simulink model "PassengerCar"  (R2019b)
settings: Solver=ode1  StartTime=0  StopTime=25  FixedStep=1.0000000000000000e-003  RelTol=1e-3
InitFcn:
  | sampleTime = str2double(get_param(bdroot, 'FixedStep'));
undefined symbols (not defined in the file or in its folder): AccPedalPos, BrakePedalPos, BrakeSwitch, DiscIntNeverNeededParam, DYNA4, EngSpd, IgnitionSwitch, InitialGear, InitialSpeed, IntendedEngTrq, LeftIndicator, MainBrakePress, MaxGear, MDL, MinGear, RefAcc, RefLane, RefLatPos, RefPath, RefPathCurv, RefSpd, RefSpdPreview, RefSpdRetrospect, RightIndicator, SteeringWheelAng, SteeringWheelTrq, UserDefinedRefValue, vm_const
libraries: UtilitiesLibrary x31, simulink x18, WheelSystemModules x13, LongitudinalControllerModules x13, LateralControllerModules x7, AnimationBusselectorModules x5, EnvironmentModules x5, BasicEngineControlModules x5, MiscellaneousControlModules x5, Animation3Modules x4, AuxiliariesModules x4, TireModules x4
(part 5 of 39)

== system PassengerCar/Traffic/TrafficOutputs ==
  Distance : Constant  Value=1000
  Distance1 : Constant  Value=0
  DistanceToVehicleOutput : Subsystem  Tag=TESIS DYNAware Interface Block  mask{NeedsUpdate=off, SignalInfo=|}
      mask SignalInfo=|
      | {
      |   "Version": "4.6",
      |   "MuxedOutputBusName": "Traffic",
      |   "MuxedInputBusName": "input",
      |   "MuxedInputSelected": false,
      |   "MuxedOutputSelected": true,
      |   "SignalData": [
      |     {
      |       "initialValue": "0.0",
      |       "name": "LeftAdjacentLaneFrontalDist[m]",
      |       "comment": "Distance of VuT to next frontal traffic object on left adjacent lane",
      |       "minString": "",
      |       "maxString": "",
      |       "width": 1,
      |       "dataType": 0,
      |       "signalType": 0,
      |       "createSignal": false,
      |       "outputName": "DistancesToVehicle.LeftAdjacentLaneFrontalDist[m]",
      |       "generateSignalAccessBlock": false,
      |       "accessId": "$(parentId).$(blockName).$(outputName)"
      |     },
      |     {
      |       "initialValue": "0.0",
      |       "name": "LeftAdjacentLaneRearDist[m]",
      |       "comment": "Distance of VuT to next rear traffic object on left adjacent lane",
      |       "minString": "",
      |       "maxString": "",
      |       "width": 1,
      |       "dataType": 0,
      |       "signalType": 0,
      |       "createSignal": false,
      |       "outputName": "DistancesToVehicle.LeftAdjacentLaneRearDist[m]",
      |       "generateSignalAccessBlock": false,
      |       "accessId": "$(parentId).$(blockName).$(outputName)"
      |     },
      |     {
      |       "initialValue": "0.0",
      |       "name": "MyLaneFrontalDist[m]",
      |       "comment": "Distance of VuT to next frontal traffic object on the same lane",
      |       "minString": "",
      |       "maxString": "",
      |       "width": 1,
      |       "dataType": 0,
      |       "signalType": 0,
      |       "createSignal": false,
      |       "outputName": "DistancesToVehicle.MyLaneFrontalDist[m]",
      |       "generateSignalAccessBlock": false,
      |       "accessId": "$(parentId).$(blockName).$(outputName)"
      |     },
      |     {
      |       "initialValue": "0.0",
      |       "name": "MyLaneRearDist[m]",
      |       "comment": "Distance of VuT to next rear traffic object on the same lane",
      |       "minString": "",
      |       "maxString": "",
      |       "width": 1,
      |       "dataType": 0,
      |       "signalType": 0,
      |       "createSignal": false,
      |       "outputName": "DistancesToVehicle.MyLaneRearDist[m]",
      |       "generateSignalAccessBlock": false,
      |       "accessId": "$(parentId).$(blockName).$(outputName)"
      |     },
      |     {
      |       "initialValue": "0.0",
      |       "name": "RightAdjacentLaneFrontalDist[m]",
      |       "comment": "Distance of VuT to next frontal traffic object on right adjacent lane",
      |       "minString": "",
      |       "maxString": "",
      |       "width": 1,
      |       "dataType": 0,
      |       "signalType": 0,
      |       "createSignal": false,
      |       "outputName": "DistancesToVehicle.RightAdjacentLaneFrontalDist[m]",
      |       "generateSignalAccessBlock": false,
      |       "accessId": "$(parentId).$(blockName).$(outputName)"
      |     },
      |     {
      |       "initialValue": "0.0",
      |       "name": "RightAdjacentLaneRearDist[m]",
      |       "comment": "Distance of VuT to next rear traffic object on right adjacent lane",
      |       "minString": "",
      |       "maxString": "",
      |       "width": 1,
      |       "dataType": 0,
      |       "signalType": 0,
      |       "createSignal": false,
      |       "outputName": "DistancesToVehicle.RightAdjacentLaneRearDist[m]",
      |       "generateSignalAccessBlock": false,
      |       "accessId": "$(parentId).$(blockName).$(outputName)"
      |     },
      |     {
      |       "initialValue": "0.0",
      |       "name": "LeftAdjacentLaneFrontalSpd[m/s]",
      |       "comment": "Longitudinal speed of next frontal traffic object on left adjacent lane",
      |       "minString": "",
      |       "maxString": "",
      |       "width": 1,
      |       "dataType": 0,
      |       "signalType": 0,
      |       "createSignal": false,
      |       "outputName": "AdjacentObjectsSpeeds.LeftAdjacentLaneFrontalSpd[m/s]",
      |       "generateSignalAccessBlock": false,
      |       "accessId": "$(parentId).$(blockName).$(outputName)"
      |     },
      |     {
      |       "initialValue": "0.0",
      |       "name": "LeftAdjacentLaneRearSpd[m/s]",
      |       "comment": "Longitudinal speed of next rear traffic object on left adjacent lane",
      |       "minString": "",
      |       "maxString": "",
      |       "width": 1,
      |       "dataType": 0,
      |       "signalType": 0,
      |       "createSignal": false,
      |       "outputName": "AdjacentObjectsSpeeds.LeftAdjacentLaneRearSpd[m/s]",
      |       "generateSignalAccessBlock": false,
      |       "accessId": "$(parentId).$(blockName).$(outputName)"
      |     },
      |     {
      |       "initialValue": "0.0",
      |       "name": "MyLaneFrontalSpd[m/s]",
      |       "comment": "Longitudinal speed of next frontal traffic object on the same lane",
      |       "minString": "",
      |       "maxString": "",
      |       "width": 1,
      |       "dataType": 0,
      |       "signalType": 0,
      |       "createSignal": false,
      |       "outputName": "AdjacentObjectsSpeeds.MyLaneFrontalSpd[m/s]",
      |       "generateSignalAccessBlock": false,
      |       "accessId": "$(parentId).$(blockName).$(outputName)"
      |     },
      |     {
      |       "initialValue": "0.0",
      |       "name": "MyLaneRearSpd[m/s]",
      |       "comment": "Longitudinal speed of next rear traffic object on the same lane",
      |       "minString": "",
      |       "maxString": "",
      |       "width": 1,
      |       "dataType": 0,
      |       "signalType": 0,
      |       "createSignal": false,
      |       "outputName": "AdjacentObjectsSpeeds.MyLaneRearSpd[m/s]",
      |       "generateSignalAccessBlock": false,
      |       "accessId": "$(parentId).$(blockName).$(outputName)"
      |     },
      |     {
      |       "initialValue": "0.0",
      |       "name": "RightAdjacentLaneFrontalSpd[m/s]",
      |       "comment": "Longitudinal speed of next frontal traffic object on right adjacent lane",
      |       "minString": "",
      |       "maxString": "",
      |       "width": 1,
      |       "dataType": 0,
      |       "signalType": 0,
      |       "createSignal": false,
      |       "outputName": "AdjacentObjectsSpeeds.RightAdjacentLaneFrontalSpd[m/s]",
      |       "generateSignalAccessBlock": false,
      |       "accessId": "$(parentId).$(blockName).$(outputName)"
      |     },
      |     {
      |       "initialValue": "0.0",
      |       "name": "RightAdjacentLaneRearSpd[m/s]",
      |       "comment": "Longitudinal speed of next rear traffic object on right adjacent lane",
      |       "minString": "",
      |       "maxString": "",
      |       "width": 1,
      |       "dataType": 0,
      |       "signalType": 0,
      |       "createSignal": false,
      |       "outputName": "AdjacentObjectsSpeeds.RightAdjacentLaneRearSpd[m/s]",
      |       "generateSignalAccessBlock": false,
      |       "accessId": "$(parentId).$(blockName).$(outputName)"
      |     }
      |   ]
      | }
      mask prompts: NeedsUpdate "Specify, if subsystem content needs to be updated"; SignalInfo "Signal Info (json)"
      mask help: DYNA4 Interface Block Version 4.6
      mask init:
      | blockName = get_param(gcbh, 'Name');
      | parentId = DYNA4.ModelHandling.AccessID.getFromHierarchy(gcbh);
      | TD.InterfaceBlock.ModelCallbacks.GenerateContent(gcb);
      settings: DeleteFcn=TD.InterfaceBlock.ModelCallbacks.CloseGUI( gcbh );  NameChangeFcn=TD.InterfaceBlock.ModelCallbacks.BlockRenamedHandler(gcbh);  OpenFcn=TD.InterfaceBlock.ModelCallbacks.OpenGUI( gcbh );  CloseFcn=TD.InterfaceBlock.ModelCallbacks.CloseGUI( gcbh );
      mask Display:
      | image('InterfaceBlock.png','center');
      | port_label('input',1, 'LeftAdjacentLaneFrontalDist[m]');
      | port_label('input',2, 'LeftAdjacentLaneRearDist[m]');
      | port_label('input',3, 'MyLaneFrontalDist[m]');
      | port_label('input',4, 'MyLaneRearDist[m]');
      | port_label('input',5, 'RightAdjacentLaneFrontalDist[m]');
      | port_label('input',6, 'RightAdjacentLaneRearDist[m]');
      | port_label('input',7, 'LeftAdjacentLaneFrontalSpd[m/s]');
      | port_label('input',8, 'LeftAdjacentLaneRearSpd[m/s]');
      | port_label('input',9, 'MyLaneFrontalSpd[m/s]');
      | port_label('input',10, 'MyLaneRearSpd[m/s]');
      | port_label('input',11, 'RightAdjacentLaneFrontalSpd[m/s]');
      | port_label('input',12, 'RightAdjacentLaneRearSpd[m/s]');
      | port_label('output',1, 'Traffic');
  Traffic : Outport  VectorParamsAs1DForOutWhenUnconnected=off
  wires:
  Distance1/1 -> DistanceToVehicleOutput/12(RightAdjacentLaneRearSpd[m/s]___UNIQUE_1), DistanceToVehicleOutput/11(RightAdjacentLaneFrontalSpd[m/s]___UNIQUE_1), DistanceToVehicleOutput/10(MyLaneRearSpd[m/s]___UNIQUE_1), DistanceToVehicleOutput/7(LeftAdjacentLaneFrontalSpd[m/s]___UNIQUE_1), DistanceToVehicleOutput/8(LeftAdjacentLaneRearSpd[m/s]___UNIQUE_1), DistanceToVehicleOutput/9(MyLaneFrontalSpd[m/s]___UNIQUE_1)
  Distance/1 -> DistanceToVehicleOutput/5(RightAdjacentLaneFrontalDist[m]___UNIQUE_1), DistanceToVehicleOutput/6(RightAdjacentLaneRearDist[m]___UNIQUE_1), DistanceToVehicleOutput/4(MyLaneRearDist[m]___UNIQUE_1), DistanceToVehicleOutput/3(MyLaneFrontalDist[m]___UNIQUE_1), DistanceToVehicleOutput/2(LeftAdjacentLaneRearDist[m]___UNIQUE_1), DistanceToVehicleOutput/1(LeftAdjacentLaneFrontalDist[m]___UNIQUE_1)
  DistanceToVehicleOutput/1(Traffic___UNIQUE_1) -> Traffic/1

== system PassengerCar/Trailer/DynaComponentInfo ==

== system PassengerCar/Vehicle/Auxiliaries ==
  fromCTRL : Inport
  fromDrivetrain : Inport  Port=2
  fromElectricalSystem : Inport  Port=3
  fromEngine : Inport  Port=4
  AuxiliariesOutput : Subsystem  Tag=TESIS DYNAware Interface Block  mask{NeedsUpdate=off, SignalInfo=|}
      mask SignalInfo=|
      | {
      |   "Version": "4.6",
      |   "MuxedOutputBusName": "Auxiliaries",
      |   "MuxedInputBusName": "input",
      |   "MuxedInputSelected": false,
      |   "MuxedOutputSelected": true,
      |   "SignalData": [
      |     {
      |       "initialValue": "0.0",
      |       "name": "GeneratorCurr[A]",
      |       "comment": "",
      |       "minString": "",
      |       "maxString": "",
      |       "width": 1,
      |       "dataType": 0,
      |       "signalType": 0,
      |       "createSignal": false,
      |       "outputName": "GeneratorCurr[A]",
      |       "generateSignalAccessBlock": false,
      |       "accessId": "$(parentId).$(blockName).$(outputName)"
      |     },
      |     {
      |       "initialValue": "0.0",
      |       "name": "GeneratorTrq[Nm]",
      |       "comment": "",
      |       "minString": "",
      |       "maxString": "",
      |       "width": 1,
      |       "dataType": 0,
      |       "signalType": 0,
      |       "createSignal": false,
      |       "outputName": "GeneratorTrq[Nm]",
      |       "generateSignalAccessBlock": false,
      |       "accessId": "$(parentId).$(blockName).$(outputName)"
      |     },
      |     {
      |       "initialValue": "0.0",
      |       "name": "GeneratorInrt[kgm^2]",
      |       "comment": "",
      |       "minString": "",
      |       "maxString": "",
      |       "width": 1,
      |       "dataType": 0,
      |       "signalType": 0,
      |       "createSignal": false,
      |       "outputName": "GeneratorInrt[kgm^2]",
      |       "generateSignalAccessBlock": false,
      |       "accessId": "$(parentId).$(blockName).$(outputName)"
      |     },
      |     {
      |       "initialValue": "0.0",
      |       "name": "StarterCurr[A]",
      |       "comment": "",
      |       "minString": "",
      |       "maxString": "",
      |       "width": 1,
      |       "dataType": 0,
      |       "signalType": 0,
      |       "createSignal": false,
      |       "outputName": "StarterCurr[A]",
      |       "generateSignalAccessBlock": false,
      |       "accessId": "$(parentId).$(blockName).$(outputName)"
      |     },
      |     {
      |       "initialValue": "0.0",
      |       "name": "StarterTrq[Nm]",
      |       "comment": "",
      |       "minString": "",
      |       "maxString": "",
      |       "width": 1,
      |       "dataType": 0,
      |       "signalType": 0,
      |       "createSignal": false,
      |       "outputName": "StarterTrq[Nm]",
      |       "generateSignalAccessBlock": false,
      |       "accessId": "$(parentId).$(blockName).$(outputName)"
      |     },
      |     {
      |       "initialValue": "0.0",
      |       "name": "StarterInrt[kgm**2]",
      |       "comment": "",
      |       "minString": "",
      |       "maxString": "",
      |       "width": 1,
      |       "dataType": 0,
      |       "signalType": 0,
      |       "createSignal": false,
      |       "outputName": "StarterInrt[kgm**2]",
      |       "generateSignalAccessBlock": false,
      |       "accessId": "$(parentId).$(blockName).$(outputName)"
      |     }
      |   ]
      | }
      mask prompts: NeedsUpdate "Specify, if subsystem content needs to be updated"; SignalInfo "Signal Info (json)"
      mask help: DYNA4 Interface Block Version 4.6
      mask init:
      | blockName = get_param(gcbh, 'Name');
      | parentId = DYNA4.ModelHandling.AccessID.getFromHierarchy(gcbh);
      | TD.InterfaceBlock.ModelCallbacks.GenerateContent(gcb);
      settings: DeleteFcn=TD.InterfaceBlock.ModelCallbacks.CloseGUI( gcbh );  NameChangeFcn=TD.InterfaceBlock.ModelCallbacks.BlockRenamedHandler(gcbh);  OpenFcn=TD.InterfaceBlock.ModelCallbacks.OpenGUI( gcbh );  CloseFcn=TD.InterfaceBlock.ModelCallbacks.CloseGUI( gcbh );
      mask Display:
      | image('InterfaceBlock.png','center');
      | port_label('input',1, 'GeneratorCurr[A]');
      | port_label('input',2, 'GeneratorTrq[Nm]');
      | port_label('input',3, 'GeneratorInrt[kgm^2]');
      | port_label('input',4, 'StarterCurr[A]');
      | port_label('input',5, 'StarterTrq[Nm]');
      | port_label('input',6, 'StarterInrt[kgm**2]');
      | port_label('output',1, 'Auxiliaries');
  DynaComponentInfo : Subsystem  Tag=DynaComponentInfo
      mask init:
      | data= get_param(gcb, 'UserData');
      settings: OpenFcn=DYNA4.ModelHandling.Component.ShowEditComponentInformationDialog(gcb);
      mask Display: disp(['Type = ', data.type, '\nGroup = ', data.group, '\nName = ', data.name ])
  Generator : Subsystem
  GeneratorTemp [K] : Constant  Value=273+80
  InputFromCTRL : Subsystem  Tag=TESIS DYNAware Interface Block  mask{NeedsUpdate=off, SignalInfo=|}
      mask SignalInfo=|
      | {
      |   "Version": "4.6",
      |   "MuxedOutputBusName": "Ctrl",
      |   "MuxedInputBusName": "fromCTRL",
      |   "MuxedInputSelected": true,
      |   "MuxedOutputSelected": false,
      |   "SignalData": [
      |     {
      |       "initialValue": "0.0",
      |       "name": "CTRL.LongitudinalControl.StarterSwitch[0;1]",
      |       "comment": "Engine starter switch",
      |       "minString": "",
      |       "maxString": "",
      |       "width": 1,
      |       "dataType": 0,
      |       "signalType": 0,
      |       "createSignal": false,
      |       "outputName": "StarterSwitch[0;1]",
      |       "generateSignalAccessBlock": false,
      |       "accessId": "$(parentId).$(blockName).$(outputName)"
      |     },
      |     {
      |       "initialValue": "0.0",
      |       "name": "CTRL.EnvironmentalConditions.AmbTemp[K]",
      |       "comment": "",
      |       "minString": "",
      |       "maxString": "",
      |       "width": 1,
      |       "dataType": 0,
      |       "signalType": 0,
      |       "createSignal": false,
      |       "outputName": "AmbTemp[K]",
      |       "generateSignalAccessBlock": false,
      |       "accessId": "$(parentId).$(blockName).$(outputName)"
      |     }
      |   ]
      | }
      mask prompts: NeedsUpdate "Specify, if subsystem content needs to be updated"; SignalInfo "Signal Info (json)"
      mask help: DYNA4 Interface Block Version 4.6
      mask init:
      | blockName = get_param(gcbh, 'Name');
      | parentId = DYNA4.ModelHandling.AccessID.getFromHierarchy(gcbh);
      | TD.InterfaceBlock.ModelCallbacks.GenerateContent(gcb);
      settings: DeleteFcn=TD.InterfaceBlock.ModelCallbacks.CloseGUI( gcbh );  NameChangeFcn=TD.InterfaceBlock.ModelCallbacks.BlockRenamedHandler(gcbh);  OpenFcn=TD.InterfaceBlock.ModelCallbacks.OpenGUI( gcbh );  CloseFcn=TD.InterfaceBlock.ModelCallbacks.CloseGUI( gcbh );
      mask Display:
      | image('InterfaceBlock.png','center');
      | port_label('input',1, 'fromCTRL');
      | port_label('output',1, 'StarterSwitch[0;1]');
      | port_label('output',2, 'AmbTemp[K]');
  InputFromDrivetrain : Subsystem  Tag=TESIS DYNAware Interface Block  mask{NeedsUpdate=off, SignalInfo=|}
      mask SignalInfo=|
      | {
      |   "Version": "4.6",
      |   "MuxedOutputBusName": "output",
      |   "MuxedInputBusName": "fromDrivetrain",
      |   "MuxedInputSelected": true,
      |   "MuxedOutputSelected": false,
      |   "SignalData": {
      |     "initialValue": "0.0",
      |     "name": "DrivetrainPhysics.EngSpd[rad/s]",
      |     "comment": "",
      |     "minString": "",
      |     "maxString": "",
      |     "width": -1,
      |     "dataType": 0,
      |     "signalType": 0,
      |     "createSignal": false,
      |     "outputName": "EngSpd[rad/s]",
      |     "generateSignalAccessBlock": false,
      |     "accessId": "$(parentId).$(blockName).$(outputName)"
      |   }
      | }
      mask prompts: NeedsUpdate "Specify, if subsystem content needs to be updated"; SignalInfo "Signal Info (json)"
      mask help: DYNA4 Interface Block Version 4.6
      mask init:
      | blockName = get_param(gcbh, 'Name');
      | parentId = DYNA4.ModelHandling.AccessID.getFromHierarchy(gcbh);
      | TD.InterfaceBlock.ModelCallbacks.GenerateContent(gcb);
      settings: DeleteFcn=TD.InterfaceBlock.ModelCallbacks.CloseGUI( gcbh );  NameChangeFcn=TD.InterfaceBlock.ModelCallbacks.BlockRenamedHandler(gcbh);  OpenFcn=TD.InterfaceBlock.ModelCallbacks.OpenGUI( gcbh );  CloseFcn=TD.InterfaceBlock.ModelCallbacks.CloseGUI( gcbh );
      mask Display:
      | image('InterfaceBlock.png','center');
      | port_label('input',1, 'fromDrivetrain');
      | port_label('output',1, 'EngSpd[rad/s]');
  InputFromElectricalSystem : Subsystem  Tag=TESIS DYNAware Interface Block  mask{NeedsUpdate=off, SignalInfo=|}
      mask SignalInfo=|
      | {
      |   "Version": "4.6",
      |   "MuxedOutputBusName": "Powernet",
      |   "MuxedInputBusName": "fromPowernet",
      |   "MuxedInputSelected": true,
      |   "MuxedOutputSelected": false,
      |   "SignalData": [
      |     {
      |       "initialValue": "0.0",
      |       "name": "GeneratorVoltage[V]",
      |       "comment": "",
      |       "minString": "",
      |       "maxString": "",
      |       "width": 1,
      |       "dataType": 0,
      |       "signalType": 0,
      |       "createSignal": false,
      |       "outputName": "GeneratorVoltage[V]",
      |       "generateSignalAccessBlock": false,
      |       "accessId": "$(parentId).$(blockName).$(outputName)"
      |     },
      |     {
      |       "initialValue": "0.0",
      |       "name": "LowVoltageBattery.LowVoltageBatteryVoltage[V]",
      |       "comment": "",
      |       "minString": "",
      |       "maxString": "",
      |       "width": 1,
      |       "dataType": 0,
      |       "signalType": 0,
      |       "createSignal": false,
      |       "outputName": "LowVoltageBatteryVoltage[V]",
      |       "generateSignalAccessBlock": false,
      |       "accessId": "$(parentId).$(blockName).$(outputName)"
      |     },
      |     {
      |       "initialValue": "0.0",
      |       "name": "StarterVoltage[V]",
      |       "comment": "",
      |       "minString": "",
      |       "maxString": "",
      |       "width": 1,
      |       "dataType": 0,
      |       "signalType": 0,
      |       "createSignal": false,
      |       "outputName": "StarterVoltage[V]",
      |       "generateSignalAccessBlock": false,
      |       "accessId": "$(parentId).$(blockName).$(outputName)"
      |     }
      |   ]
      | }
      mask prompts: NeedsUpdate "Specify, if subsystem content needs to be updated"; SignalInfo "Signal Info (json)"
      mask help: DYNA4 Interface Block Version 4.6
      mask init:
      | blockName = get_param(gcbh, 'Name');
      | parentId = DYNA4.ModelHandling.AccessID.getFromHierarchy(gcbh);
      | TD.InterfaceBlock.ModelCallbacks.GenerateContent(gcb);
      settings: DeleteFcn=TD.InterfaceBlock.ModelCallbacks.CloseGUI( gcbh );  NameChangeFcn=TD.InterfaceBlock.ModelCallbacks.BlockRenamedHandler(gcbh);  OpenFcn=TD.InterfaceBlock.ModelCallbacks.OpenGUI( gcbh );  CloseFcn=TD.InterfaceBlock.ModelCallbacks.CloseGUI( gcbh );
      mask Display:
      | image('InterfaceBlock.png','center');
      | port_label('input',1, 'fromPowernet');
      | port_label('output',1, 'GeneratorVoltage[V]');
      | port_label('output',2, 'LowVoltageBatteryVoltage[V]');
      | port_label('output',3, 'StarterVoltage[V]');
  LoadResponse [s] : Constant  Value=3
  SimpleEnergyManagement : Subsystem
  Starter : Subsystem
  Terminator_6 : Terminator
  TraceMarker : UtilitiesLibrary/DYNA4 Trace Marker  Tag=DYNA4_TRACE_MARKER  SettingType=Standard  PrefixModelBlockID=on  PrefixRootSignalName=off  NamePattern='$(modelBlockID).$(rootSignalName)'
  Auxiliaries : Outport  VectorParamsAs1DForOutWhenUnconnected=off
  wires:
  InputFromElectricalSystem/3(StarterVoltage[V]___UNIQUE_1) -> Starter/1(StarterVoltage [V])
  Generator/1(Curr [A]) -> AuxiliariesOutput/1(GeneratorCurr[A]___UNIQUE_1)
  Generator/2(Trq [Nm]) -> AuxiliariesOutput/2(GeneratorTrq[Nm]___UNIQUE_1)
  Generator/3(Inrt [kgm**2]) -> AuxiliariesOutput/3(GeneratorInrt[kgm^2]___UNIQUE_1)
  InputFromCTRL/1(StarterSwitch[0;1]___UNIQUE_1) -> Starter/3(StarterSwitch [0;1]), SimpleEnergyManagement/1(StarterSwitch [0;1])
  Starter/1(StarterCurr [A]) -> AuxiliariesOutput/4(StarterCurr[A]___UNIQUE_1)
  InputFromCTRL/2(AmbTemp[K]___UNIQUE_1) -> Starter/4(Temp [K])
  LoadResponse [s]/1 -> Generator/4(LRTime [s])
  SimpleEnergyManagement/1(RefVoltage [V]) -> Generator/3(RefVoltage [V])
  GeneratorTemp [K]/1 -> Generator/5(Temp [K])
  Starter/2(StarterTrq [Nm]) -> AuxiliariesOutput/5(StarterTrq[Nm]___UNIQUE_1)
  fromDrivetrain/1 -> InputFromDrivetrain/1(fromDrivetrain)
  fromEngine/1 -> Terminator_6/1
  fromElectricalSystem/1 -> InputFromElectricalSystem/1(fromPowernet)
  InputFromDrivetrain/1(EngSpd[rad/s]) -> Generator/1(EngSpd [rad/s]), Starter/2(EngSpd [rad/s])
  InputFromElectricalSystem/2(LowVoltageBatteryVoltage[V]___UNIQUE_1) -> Generator/6(BattVoltage [V])
  fromCTRL/1 -> InputFromCTRL/1(fromCTRL)
  AuxiliariesOutput/1(Auxiliaries___UNIQUE_1) -> TraceMarker/1, Auxiliaries/1
  InputFromElectricalSystem/1(GeneratorVoltage[V]___UNIQUE_1) -> Generator/2(GeneratorVoltage [V])
  Starter/3(StarterInrt [kgm**2]) -> AuxiliariesOutput/6(StarterInrt[kgm**2]___UNIQUE_1)

== system PassengerCar/Vehicle/BrakeSystem ==
  fromCTRL : Inport
  fromChassis : Inport  Port=2
  fromEngine : Inport  Port=3
  fromWheelSystem : Inport  Port=4
  BrakeControlCoordinator : ControllerLibrary/BrakeControlCoordinator  SystemSampleTime=-1  Latency=0  AutoFrameSizeCalculation=off
  BrakeSystemControlUnit : Subsystem
  BrakeSystemOutputs : Subsystem  Tag=TESIS DYNAware Interface Block  mask{NeedsUpdate=off, SignalInfo=|}
      mask SignalInfo=|
      | {
      |   "Version": "4.6",
      |   "MuxedOutputBusName": "BrakeSystem",
      |   "MuxedInputBusName": "",
      |   "MuxedInputSelected": false,
      |   "MuxedOutputSelected": true,
      |   "SignalData": [
      |     {
      |       "initialValue": "0.0",
      |       "name": "BrakeSystemPhysics",
      |       "comment": "",
      |       "minString": "",
      |       "maxString": "",
      |       "width": -1,
      |       "dataType": 0,
      |       "signalType": 1,
      |       "createSignal": false,
      |       "outputName": "BrakeSystemPhysics",
      |       "generateSignalAccessBlock": false,
      |       "accessId": "$(parentId).$(blockName).$(outputName)"
      |     },
      |     {
      |       "initialValue": "0.0",
      |       "name": "BrakeSystemControlUnitInfo",
      |       "comment": "",
      |       "minString": "",
      |       "maxString": "",
      |       "width": -1,
      |       "dataType": 0,
      |       "signalType": 1,
      |       "createSignal": false,
      |       "outputName": "BrakeSystemControlUnitInfo",
      |       "generateSignalAccessBlock": false,
      |       "accessId": "$(parentId).$(blockName).$(outputName)"
      |     }
      |   ]
      | }
      mask prompts: NeedsUpdate "Specify, if subsystem content needs to be updated"; SignalInfo "Signal Info (json)"
      mask help: DYNA4 Interface Block Version 4.6
      mask init:
      | blockName = get_param(gcbh, 'Name');
      | parentId = DYNA4.ModelHandling.AccessID.getFromHierarchy(gcbh);
      | TD.InterfaceBlock.ModelCallbacks.GenerateContent(gcb);
      settings: DeleteFcn=TD.InterfaceBlock.ModelCallbacks.CloseGUI( gcbh );  NameChangeFcn=TD.InterfaceBlock.ModelCallbacks.BlockRenamedHandler(gcbh);  OpenFcn=TD.InterfaceBlock.ModelCallbacks.OpenGUI( gcbh );  CloseFcn=TD.InterfaceBlock.ModelCallbacks.CloseGUI( gcbh );
      mask Display:
      | image('InterfaceBlock.png','center');
      | port_label('input',1, 'BrakeSystemPhysics');
      | port_label('input',2, 'BrakeSystemControlUnitInfo');
      | port_label('output',1, 'BrakeSystem');
  BrakeSystemPhysics : Subsystem
  BrakeSystemPhysicsOutput : Subsystem  Tag=TESIS DYNAware Interface Block  mask{NeedsUpdate=off, SignalInfo=|}
      mask SignalInfo=|
      | {
      |   "Version": "4.6",
      |   "MuxedOutputBusName": "BrakeSystem",
      |   "MuxedInputBusName": "input",
      |   "MuxedInputSelected": false,
      |   "MuxedOutputSelected": true,
      |   "SignalData": [
      |     {
      |       "initialValue": "0.0",
      |       "name": "MaxMainBrakePress[Pa]",
      |       "comment": "",
      |       "minString": "",
      |       "maxString": "",
      |       "width": 1,
      |       "dataType": 0,
      |       "signalType": 0,
      |       "createSignal": false,
      |       "outputName": "MaxMainBrakePress[Pa]",
      |       "generateSignalAccessBlock": false,
      |       "accessId": "$(parentId).$(blockName).$(outputName)"
      |     },
      |     {
      |       "initialValue": "0.0",
      |       "name": "MainBrakePress[Pa]",
      |       "comment": "",
      |       "minString": "",
      |       "maxString": "",
      |       "width": 1,
      |       "dataType": 0,
      |       "signalType": 0,
      |       "createSignal": false,
      |       "outputName": "MainBrakePress[Pa]",
      |       "generateSignalAccessBlock": false,
      |       "accessId": "$(parentId).$(blockName).$(outputName)"
      |     },
      |     {
      |       "initialValue": "",
      |       "name": "FrontLeftWheelBrakePress[Pa]",
      |       "comment": "",
      |       "minString": "",
      |       "maxString": "",
      |       "width": -1,
      |       "dataType": 0,
      |       "signalType": 0,
      |       "createSignal": false,
      |       "outputName": "FrontLeftWheelBrakePress[Pa]",
      |       "generateSignalAccessBlock": false,
      |       "accessId": "$(parentId).$(blockName).$(outputName)"
      |     },
      |     {
      |       "initialValue": "",
      |       "name": "FrontRightWheelBrakePress[Pa]",
      |       "comment": "",
      |       "minString": "",
      |       "maxString": "",
      |       "width": -1,
      |       "dataType": 0,
      |       "signalType": 0,
      |       "createSignal": false,
      |       "outputName": "FrontRightWheelBrakePress[Pa]",
      |       "generateSignalAccessBlock": false,
      |       "accessId": "$(parentId).$(blockName).$(outputName)"
      |     },
      |     {
      |       "initialValue": "",
      |       "name": "RearLeftWheelBrakePress[Pa]",
      |       "comment": "",
      |       "minString": "",
      |       "maxString": "",
      |       "width": -1,
      |       "dataType": 0,
      |       "signalType": 0,
      |       "createSignal": false,
      |       "outputName": "RearLeftWheelBrakePress[Pa]",
      |       "generateSignalAccessBlock": false,
      |       "accessId": "$(parentId).$(blockName).$(outputName)"
      |     },
      |     {
      |       "initialValue": "",
      |       "name": "RearRightWheelBrakePress[Pa]",
      |       "comment": "",
      |       "minString": "",
      |       "maxString": "",
      |       "width": -1,
      |       "dataType": 0,
      |       "signalType": 0,
      |       "createSignal": false,
      |       "outputName": "RearRightWheelBrakePress[Pa]",
      |       "generateSignalAccessBlock": false,
      |       "accessId": "$(parentId).$(blockName).$(outputName)"
      |     },
      |     {
      |       "initialValue": "",
      |       "name": "Rear2LeftWheelBrakePress[Pa]",
      |       "comment": "",
      |       "minString": "",
      |       "maxString": "",
      |       "width": -1,
      |       "dataType": 0,
      |       "signalType": 0,
      |       "createSignal": false,
      |       "outputName": "Rear2LeftWheelBrakePress[Pa]",
      |       "generateSignalAccessBlock": false,
      |       "accessId": "$(parentId).$(blockName).$(outputName)"
      |     },
      |     {
      |       "initialValue": "",
      |       "name": "Rear2RightWheelBrakePress[Pa]",
      |       "comment": "",
      |       "minString": "",
      |       "maxString": "",
      |       "width": -1,
      |       "dataType": 0,
      |       "signalType": 0,
      |       "createSignal": false,
      |       "outputName": "Rear2RightWheelBrakePress[Pa]",
      |       "generateSignalAccessBlock": false,
      |       "accessId": "$(parentId).$(blockName).$(outputName)"
      |     },
      |     {
      |       "initialValue": "",
      |       "name": "Rear3LeftWheelBrakePress[Pa]",
      |       "comment": "",
      |       "minString": "",
      |       "maxString": "",
      |       "width": -1,
      |       "dataType": 0,
      |       "signalType": 0,
      |       "createSignal": false,
      |       "outputName": "Rear3LeftWheelBrakePress[Pa]",
      |       "generateSignalAccessBlock": false,
      |       "accessId": "$(parentId).$(blockName).$(outputName)"
      |     },
      |     {
      |       "initialValue": "",
      |       "name": "Rear3RightWheelBrakePress[Pa]",
      |       "comment": "",
      |       "minString": "",
      |       "maxString": "",
      |       "width": -1,
      |       "dataType": 0,
      |       "signalType": 0,
      |       "createSignal": false,
      |       "outputName": "Rear3RightWheelBrakePress[Pa]",
      |       "generateSignalAccessBlock": false,
      |       "accessId": "$(parentId).$(blockName).$(outputName)"
      |     },
      |     {
      |       "initialValue": "0.0",
      |       "name": "WheelBrakePressSource[-]",
      |       "comment": "",
      |       "minString": "",
      |       "maxString": "",
      |       "width": 1,
      |       "dataType": 0,
      |       "signalType": 0,
      |       "createSignal": false,
      |       "outputName": "WheelBrakePressSource[-]",
      |       "generateSignalAccessBlock": false,
      |       "accessId": "$(parentId).$(blockName).$(outputName)"
      |     }
      |   ]
      | }
      mask prompts: NeedsUpdate "Specify, if subsystem content needs to be updated"; SignalInfo "Signal Info (json)"
      mask help: DYNA4 Interface Block Version 4.6
      mask init:
      | blockName = get_param(gcbh, 'Name');
      | parentId = DYNA4.ModelHandling.AccessID.getFromHierarchy(gcbh);
      | TD.InterfaceBlock.ModelCallbacks.GenerateContent(gcb);
      settings: DeleteFcn=TD.InterfaceBlock.ModelCallbacks.CloseGUI( gcbh );  NameChangeFcn=TD.InterfaceBlock.ModelCallbacks.BlockRenamedHandler(gcbh);  OpenFcn=TD.InterfaceBlock.ModelCallbacks.OpenGUI( gcbh );  CloseFcn=TD.InterfaceBlock.ModelCallbacks.CloseGUI( gcbh );
      mask Display:
      | image('InterfaceBlock.png','center');
      | port_label('input',1, 'MaxMainBrakePress[Pa]');
      | port_label('input',2, 'MainBrakePress[Pa]');
      | port_label('input',3, 'FrontLeftWheelBrakePress[Pa]');
      | port_label('input',4, 'FrontRightWheelBrakePress[Pa]');
      | port_label('input',5, 'RearLeftWheelBrakePress[Pa]');
      | port_label('input',6, 'RearRightWheelBrakePress[Pa]');
      | port_label('input',7, 'Rear2LeftWheelBrakePress[Pa]');
      | port_label('input',8, 'Rear2RightWheelBrakePress[Pa]');
      | port_label('input',9, 'Rear3LeftWheelBrakePress[Pa]');
      | port_label('input',10, 'Rear3RightWheelBrakePress[Pa]');
      | port_label('input',11, 'WheelBrakePressSource[-]');
      | port_label('output',1, 'BrakeSystem');
  Bus Selector : BusSelector  OutputSignals=WheelBrakePressActive[0;1],ControlUnit  OutputAsBus=on
  Bus Selector1 : BusSelector  OutputSignals=MaxMainBrakePress[Pa],MainBrakePress[Pa]
  Bus Selector2 : BusSelector  OutputSignals=FrontLeftWheelBrakePress[Pa],FrontRightWheelBrakePress[Pa],RearLeftWheelBrakePress[Pa],RearRightWheelBrakePress[Pa],Rear2LeftWheelBrakePress[Pa],Rear2RightWheelBrakePress[Pa],Rear3LeftWheelBrakePress[Pa],Rear3RightWheelBrakePress[Pa]
  DynaComponentInfo : Subsystem  Tag=DynaComponentInfo
      mask init:
      | data= get_param(gcb, 'UserData');
      settings: OpenFcn=DYNA4.ModelHandling.Component.ShowEditComponentInformationDialog(gcb);
      mask Display: disp(['Type = ', data.type, '\nGroup = ', data.group, '\nName = ', data.name ])
  Memory : Memory  InheritSampleTime=on
  Signal Prioritizer : Subsystem  Tag=SignalPrioritizer  mask(SignalPrioritizer){SignalSource={'BrakeControlCoordinator', 'BrakeSystemControlUnit', 'BrakeSystemPhysics'}, SourcesActiveSignal='WheelBrakePressActive[0;1]', ControlSignals={'FrontLeftWheelBrakePress[Pa]', 'FrontRightWheelBrakePress[Pa]', 'RearLeftWheelBrakePress[Pa]', 'RearRightWheelBrakePress[Pa]', 'Rear2LeftWheelBrakePress[Pa]', 'Rear2RightWheelBrakePress[Pa]', 'Rear3LeftWheelBrakePress[Pa]', 'Rear3RightWheelBrakePress[Pa]'}, SignalPrioritizerVersion=2.0}
      mask prompts: SignalSource "Signal sources"; SourcesActiveSignal "Source's active signal"; ControlSignals "Control signals"; SignalPrioritizerVersion "DYNA4 Signal Prioritizer Version"
      mask help: Feed through signals from a specific source depending on it's priority and whether it is currently active.
      settings: CopyFcn=set_param(gcb,'LinkStatus','none');
      mask Help: eval('dm_rmi_set_help_context_id(''DriverAssistanceSystemsModules/SignalPrioritizer'');');
      mask Callback SignalSource: TD.UtilitiesLibrary.SignalPrioritizer.GenerateContent(gcb)
      mask Callback SourcesActiveSignal: TD.UtilitiesLibrary.SignalPrioritizer.GenerateContent(gcb)
      mask Callback ControlSignals: TD.UtilitiesLibrary.SignalPrioritizer.GenerateContent(gcb)
      mask DialogControl SignalSource Tooltip: Cell array of inport names, the order defines their priority
      mask DialogControl SourcesActiveSignal Tooltip: Name of the signal that specifies whether a source is currently active
      mask DialogControl ControlSignals Tooltip: Cell array containing the names of signals passed through
  Terminator_3 : Terminator
  TraceMarker : UtilitiesLibrary/DYNA4 Trace Marker  Tag=DYNA4_TRACE_MARKER  SettingType=Standard  PrefixModelBlockID=on  PrefixRootSignalName=off  NamePattern='$(modelBlockID).$(rootSignalName)'
  BrakeSystem : Outport  VectorParamsAs1DForOutWhenUnconnected=off
  wires:
  Memory/1 -> BrakeSystemPhysicsOutput/1(MaxMainBrakePress[Pa]___UNIQUE_1)
  fromEngine/1 -> Terminator_3/1
  Bus Selector1/2 -> BrakeSystemPhysicsOutput/2(MainBrakePress[Pa]___UNIQUE_1)  "<MainBrakePress[Pa]>"
  Bus Selector2/2 -> BrakeSystemPhysicsOutput/4(FrontRightWheelBrakePress[Pa]___UNIQUE_1)  "<FrontRightWheelBrakePress[Pa]>"
  Signal Prioritizer/1(ControlSignals) -> Bus Selector2/1
  Bus Selector2/6 -> BrakeSystemPhysicsOutput/8(Rear2RightWheelBrakePress[Pa]___UNIQUE_1)  "<Rear2RightWheelBrakePress[Pa]>"
  BrakeControlCoordinator/1 -> Signal Prioritizer/1(BrakeControlCoordinator)
  Signal Prioritizer/2(SelectedInput) -> BrakeSystemPhysicsOutput/11(WheelBrakePressSource[-]___UNIQUE_1)
  fromWheelSystem/1 -> BrakeSystemControlUnit/3(fromWheelSystem)
  Bus Selector/1 -> BrakeSystemOutputs/2(BrakeSystemControlUnitInfo___UNIQUE_1)
  Bus Selector2/1 -> BrakeSystemPhysicsOutput/3(FrontLeftWheelBrakePress[Pa]___UNIQUE_1)  "<FrontLeftWheelBrakePress[Pa]>"
  Bus Selector2/3 -> BrakeSystemPhysicsOutput/5(RearLeftWheelBrakePress[Pa]___UNIQUE_1)  "<RearLeftWheelBrakePress[Pa]>"
  Bus Selector2/5 -> BrakeSystemPhysicsOutput/7(Rear2LeftWheelBrakePress[Pa]___UNIQUE_1)  "<Rear2LeftWheelBrakePress[Pa]>"
  Bus Selector2/7 -> BrakeSystemPhysicsOutput/9(Rear3LeftWheelBrakePress[Pa]___UNIQUE_1)  "<Rear3LeftWheelBrakePress[Pa]>"
  fromCTRL/1 -> BrakeSystemPhysics/2(fromCTRL), BrakeSystemControlUnit/2(fromCTRL), BrakeControlCoordinator/1
  BrakeSystemPhysics/1(BrakeSystemPhysics) -> Bus Selector1/1, Signal Prioritizer/3(BrakeSystemPhysics), BrakeSystemControlUnit/1(fromBrakeSystemPhysics)
  fromChassis/1 -> BrakeSystemControlUnit/4(fromChassis)
  BrakeControlCoordinator/2 -> BrakeSystemPhysics/1(fromBrakeControlCoordinator)
  BrakeSystemOutputs/1(BrakeSystem___UNIQUE_1) -> TraceMarker/1, BrakeSystem/1
  Bus Selector2/8 -> BrakeSystemPhysicsOutput/10(Rear3RightWheelBrakePress[Pa]___UNIQUE_1)  "<Rear3RightWheelBrakePress[Pa]>"
  BrakeSystemControlUnit/1(BrakeSystemControlUnit) -> BrakeSystemPhysics/3(fromBrakeSystemControlUnit), Signal Prioritizer/2(BrakeSystemControlUnit), Bus Selector/1
  Bus Selector1/1 -> Memory/1  "<MaxMainBrakePress[Pa]>"
  Bus Selector2/4 -> BrakeSystemPhysicsOutput/6(RearRightWheelBrakePress[Pa]___UNIQUE_1)  "<RearRightWheelBrakePress[Pa]>"
  BrakeSystemPhysicsOutput/1(BrakeSystem___UNIQUE_1) -> BrakeSystemOutputs/1(BrakeSystemPhysics___UNIQUE_1)

== system PassengerCar/Vehicle/Chassis ==
  fromCTRL : Inport
  fromTrailer : Inport  Port=2
  fromEngine : Inport  Port=3
  fromWheelSystem : Inport  Port=4
  ComponentSpecificChassisInputs : Subsystem
  DynaComponentInfo : Subsystem  Tag=DynaComponentInfo
      mask init:
      | data= get_param(gcb, 'UserData');
      settings: OpenFcn=DYNA4.ModelHandling.Component.ShowEditComponentInformationDialog(gcb);
      mask Display: disp(['Type = ', data.type, '\nGroup = ', data.group, '\nName = ', data.name ])
  MultiBodyChassis : ChassisModules/MultiBodyChassis  Tag=vedynaChassisMask  local_comp_inst=1  system_comp_inst=1  DATA_NODE=MDL.Vehicle.Chassis  sample_time=-1
  TraceMarker : UtilitiesLibrary/DYNA4 Trace Marker  Tag=DYNA4_TRACE_MARKER  SettingType=Standard  PrefixModelBlockID=on  PrefixRootSignalName=off  NamePattern='$(modelBlockID).$(rootSignalName)'
  Chassis : Outport  VectorParamsAs1DForOutWhenUnconnected=off
  wires:
  fromEngine/1 -> MultiBodyChassis/3
  fromTrailer/1 -> MultiBodyChassis/2
  fromWheelSystem/1 -> MultiBodyChassis/4
  fromCTRL/1 -> MultiBodyChassis/1
  MultiBodyChassis/1 -> TraceMarker/1, Chassis/1
  ComponentSpecificChassisInputs/1(SteeringInputs) -> MultiBodyChassis/5
  ComponentSpecificChassisInputs/2(ActuatedTrackRodInputs) -> MultiBodyChassis/6

== system PassengerCar/Vehicle/CoolingSystem ==
  fromCTRL : Inport
  fromChassis : Inport  Port=2
  fromEngine : Inport  Port=3
  fromDrivetrain : Inport  Port=4
  fromElectricalSystem : Inport  Port=5
  fromEnvironment : Inport  Port=6
  CoolingSystemOutput : Subsystem  Tag=TESIS DYNAware Interface Block  mask{NeedsUpdate=off, SignalInfo=|}
      mask SignalInfo=|
      | {
      |   "Version": "4.6",
      |   "MuxedOutputBusName": "CoolingSystem",
      |   "MuxedInputBusName": "input",
      |   "MuxedInputSelected": false,
      |   "MuxedOutputSelected": true,
      |   "SignalData": {
      |     "initialValue": "0.0",
      |     "name": "NoCoolingSystem",
      |     "comment": "",
      |     "minString": "",
      |     "maxString": "",
      |     "width": 1,
      |     "dataType": 0,
      |     "signalType": 0,
      |     "createSignal": false,
      |     "outputName": "NoCoolingSystem",
      |     "generateSignalAccessBlock": false,
      |     "accessId": "$(parentId).$(blockName).$(outputName)"
      |   }
      | }
      mask prompts: NeedsUpdate "Specify, if subsystem content needs to be updated"; SignalInfo "Signal Info (json)"
      mask help: DYNA4 Interface Block Version 4.6
      mask init:
      | blockName = get_param(gcbh, 'Name');
      | parentId = DYNA4.ModelHandling.AccessID.getFromHierarchy(gcbh);
      | TD.InterfaceBlock.ModelCallbacks.GenerateContent(gcb);
      settings: DeleteFcn=TD.InterfaceBlock.ModelCallbacks.CloseGUI( gcbh );  NameChangeFcn=TD.InterfaceBlock.ModelCallbacks.BlockRenamedHandler(gcbh);  OpenFcn=TD.InterfaceBlock.ModelCallbacks.OpenGUI( gcbh );  CloseFcn=TD.InterfaceBlock.ModelCallbacks.CloseGUI( gcbh );
      mask Display:
      | image('InterfaceBlock.png','center');
      | port_label('input',1, 'NoCoolingSystem');
      | port_label('output',1, 'CoolingSystem');
  DynaComponentInfo : Subsystem  Tag=DynaComponentInfo
      mask init:
      | data = get_param(gcb, 'UserData');
      settings: OpenFcn=DYNA4.ModelHandling.Component.ShowEditComponentInformationDialog(gcb);
      mask Display: disp(['Type = ', data.type, '\nGroup = ', data.group, '\nName = ', data.name ])
  NoCoolingSystem : Constant
  Terminator{,1..5} (6 alike) : Terminator
  CoolingSystem : Outport  VectorParamsAs1DForOutWhenUnconnected=off
  wires:
  fromEnvironment/1 -> Terminator5/1
  fromCTRL/1 -> Terminator4/1
  fromElectricalSystem/1 -> Terminator3/1
  fromDrivetrain/1 -> Terminator2/1
  fromEngine/1 -> Terminator1/1
  fromChassis/1 -> Terminator/1
  NoCoolingSystem/1 -> CoolingSystemOutput/1(NoCoolingSystem___UNIQUE_1)
  CoolingSystemOutput/1(CoolingSystem___UNIQUE_1) -> CoolingSystem/1

== system PassengerCar/Vehicle/Drivetrain ==
  fromCTRL : Inport
  fromAuxiliaries : Inport  Port=2
  fromElectricalSystem : Inport  Port=3
  fromEngine : Inport  Port=4
  fromWheelSystem : Inport  Port=5
  DYNA4 Trace Marker : UtilitiesLibrary/DYNA4 Trace Marker  Tag=DYNA4_TRACE_MARKER  SettingType=Standard  PrefixModelBlockID=on  PrefixRootSignalName=off  NamePattern='$(modelBlockID).$(rootSignalName)'
  DrivetrainControlUnit : Subsystem  Tag=COMPONENT_ENGINE
  DrivetrainOutputs : Subsystem  Tag=TESIS DYNAware Interface Block  mask{NeedsUpdate=off, SignalInfo=|}
      mask SignalInfo=|
      | {
      |   "Version": "4.6",
      |   "MuxedOutputBusName": "Drivetrain",
      |   "MuxedInputBusName": "",
      |   "MuxedInputSelected": false,
      |   "MuxedOutputSelected": true,
      |   "SignalData": [
      |     {
      |       "initialValue": "0.0",
      |       "name": "DrivetrainPhysics",
      |       "comment": "",
      |       "minString": "",
      |       "maxString": "",
      |       "width": -1,
      |       "dataType": 0,
      |       "signalType": 1,
      |       "createSignal": false,
      |       "outputName": "DrivetrainPhysics",
      |       "generateSignalAccessBlock": false,
      |       "accessId": "$(parentId).$(blockName).$(outputName)"
      |     },
      |     {
      |       "initialValue": "0.0",
      |       "name": "DrivetrainControlUnit",
      |       "comment": "",
      |       "minString": "",
      |       "maxString": "",
      |       "width": -1,
      |       "dataType": 0,
      |       "signalType": 1,
      |       "createSignal": false,
      |       "outputName": "DrivetrainControlUnit",
      |       "generateSignalAccessBlock": false,
      |       "accessId": "$(parentId).$(blockName).$(outputName)"
      |     }
      |   ]
      | }
      mask prompts: NeedsUpdate "Specify, if subsystem content needs to be updated"; SignalInfo "Signal Info (json)"
      mask help: DYNA4 Interface Block Version 4.6
      mask init:
      | blockName = get_param(gcbh, 'Name');
      | parentId = DYNA4.ModelHandling.AccessID.getFromHierarchy(gcbh);
      | TD.InterfaceBlock.ModelCallbacks.GenerateContent(gcb);
      settings: DeleteFcn=TD.InterfaceBlock.ModelCallbacks.CloseGUI( gcbh );  NameChangeFcn=TD.InterfaceBlock.ModelCallbacks.BlockRenamedHandler(gcbh);  OpenFcn=TD.InterfaceBlock.ModelCallbacks.OpenGUI( gcbh );  CloseFcn=TD.InterfaceBlock.ModelCallbacks.CloseGUI( gcbh );
      mask Display:
      | image('InterfaceBlock.png','center');
      | port_label('input',1, 'DrivetrainPhysics');
      | port_label('input',2, 'DrivetrainControlUnit');
      | port_label('output',1, 'Drivetrain');
  DrivetrainPhysics : Subsystem  Tag=COMPONENT_ENGINE
  DynaComponentInfo : Subsystem  Tag=DynaComponentInfo
      mask init:
      | data= get_param(gcb, 'UserData');
      settings: OpenFcn=DYNA4.ModelHandling.Component.ShowEditComponentInformationDialog(gcb);
      mask Display: disp(['Type = ', data.type, '\nGroup = ', data.group, '\nName = ', data.name ])
  Drivetrain : Outport  VectorParamsAs1DForOutWhenUnconnected=off
  wires:
  DrivetrainPhysics/1(DrivetrainPhysics) -> DrivetrainControlUnit/1(fromDrivetrainPhysics), DrivetrainOutputs/1(DrivetrainPhysics___UNIQUE_1)
  fromElectricalSystem/1 -> DrivetrainPhysics/4(fromElectricalSystem)
  fromAuxiliaries/1 -> DrivetrainPhysics/3(fromAuxiliaries)
  DrivetrainControlUnit/1(DrivetrainControlUnit) -> DrivetrainPhysics/1(fromDrivetrainControlUnit), DrivetrainOutputs/2(DrivetrainControlUnit___UNIQUE_1)
  fromCTRL/1 -> DrivetrainPhysics/2(fromCTRL), DrivetrainControlUnit/2(fromCTRL)
  DrivetrainOutputs/1(Drivetrain___UNIQUE_1) -> Drivetrain/1, DYNA4 Trace Marker/1
  fromWheelSystem/1 -> DrivetrainPhysics/6(fromWheelSystem)
  fromEngine/1 -> DrivetrainPhysics/5(fromEngine), DrivetrainControlUnit/3(fromEngine)

== system PassengerCar/Vehicle/DynaComponentInfo ==

== system PassengerCar/Vehicle/ElectricalSystem ==
  fromCTRL : Inport
  fromAuxiliaries : Inport  Port=2
  fromDrivetrain : Inport  Port=3
  fromEngine : Inport  Port=4
  DynaComponentInfo : Subsystem  Tag=DynaComponentInfo
      mask init:
      | data= get_param(gcb, 'UserData');
      settings: OpenFcn=DYNA4.ModelHandling.Component.ShowEditComponentInformationDialog(gcb);
      mask Display: disp(['Type = ', data.type, '\nGroup = ', data.group, '\nName = ', data.name ])
  ElectricalSystemOutput : Subsystem  Tag=TESIS DYNAware Interface Block  mask{NeedsUpdate=off, SignalInfo=|}
      mask SignalInfo=|
      | {
      |   "Version": "4.6",
      |   "MuxedOutputBusName": "ElectricalSystem",
      |   "MuxedInputBusName": "input",
      |   "MuxedInputSelected": false,
      |   "MuxedOutputSelected": true,
      |   "SignalData": [
      |     {
      |       "initialValue": "0.0",
      |       "name": "LowVoltageBattery",
      |       "comment": "Voltage level of low voltage battery",
      |       "minString": "",
      |       "maxString": "",
      |       "width": -1,
      |       "dataType": 0,
      |       "signalType": 1,
      |       "createSignal": false,
      |       "outputName": "LowVoltageBattery",
      |       "generateSignalAccessBlock": false,
      |       "accessId": "$(parentId).$(blockName).$(outputName)"
      |     },
      |     {
      |       "initialValue": "0.0",
      |       "name": "StarterVoltage[V]",
      |       "comment": "Voltage level of starter",
      |       "minString": "",
      |       "maxString": "",
      |       "width": 1,
      |       "dataType": 0,
      |       "signalType": 0,
      |       "createSignal": false,
      |       "outputName": "StarterVoltage[V]",
      |       "generateSignalAccessBlock": false,
      |       "accessId": "$(parentId).$(blockName).$(outputName)"
      |     },
      |     {
      |       "initialValue": "0.0",
      |       "name": "GeneratorVoltage[V]",
      |       "comment": "Voltage level of generator",
      |       "minString": "",
      |       "maxString": "",
      |       "width": 1,
      |       "dataType": 0,
      |       "signalType": 0,
      |       "createSignal": false,
      |       "outputName": "GeneratorVoltage[V]",
      |       "generateSignalAccessBlock": false,
      |       "accessId": "$(parentId).$(blockName).$(outputName)"
      |     }
      |   ]
      | }
      mask prompts: NeedsUpdate "Specify, if subsystem content needs to be updated"; SignalInfo "Signal Info (json)"
      mask help: DYNA4 Interface Block Version 4.6
      mask init:
      | blockName = get_param(gcbh, 'Name');
      | parentId = DYNA4.ModelHandling.AccessID.getFromHierarchy(gcbh);
      | TD.InterfaceBlock.ModelCallbacks.GenerateContent(gcb);
      settings: DeleteFcn=TD.InterfaceBlock.ModelCallbacks.CloseGUI( gcbh );  NameChangeFcn=TD.InterfaceBlock.ModelCallbacks.BlockRenamedHandler(gcbh);  OpenFcn=TD.InterfaceBlock.ModelCallbacks.OpenGUI( gcbh );  CloseFcn=TD.InterfaceBlock.ModelCallbacks.CloseGUI( gcbh );
      mask Display:
      | image('InterfaceBlock.png','center');
      | port_label('input',1, 'LowVoltageBattery');
      | port_label('input',2, 'StarterVoltage[V]');
      | port_label('input',3, 'GeneratorVoltage[V]');
      | port_label('output',1, 'ElectricalSystem');
  LowVoltageBatteryInitialSOC : LookupTableModules/ConstantSOC  DATA_NODE=MDL.Vehicle.ElectricalSystem.LowVoltageBatteryInitialSOC  SOC=MDL.Vehicle.ElectricalSystem.LowVoltageBatteryInitialSOC.SOC
  LowVoltageBatteryOutput : Subsystem  Tag=TESIS DYNAware Interface Block  mask{NeedsUpdate=off, SignalInfo=|}
      mask SignalInfo=|
      | {
      |   "Version": "4.6",
      |   "MuxedOutputBusName": "LowVoltageBattery",
      |   "MuxedInputBusName": "input",
      |   "MuxedInputSelected": false,
      |   "MuxedOutputSelected": true,
      |   "SignalData": [
      |     {
      |       "initialValue": "0.0",
      |       "name": "LowVoltageBatteryVoltage[V]",
      |       "comment": "RMS voltage at inverter output",
      |       "minString": "",
      |       "maxString": "",
      |       "width": 1,
      |       "dataType": 0,
      |       "signalType": 0,
      |       "createSignal": false,
      |       "outputName": "LowVoltageBatteryVoltage[V]",
      |       "generateSignalAccessBlock": false,
      |       "accessId": "$(parentId).$(blockName).$(outputName)"
      |     },
      |     {
      |       "initialValue": "0.0",
      |       "name": "LowVoltageBatterySOC[0_1]",
      |       "comment": "Current at inverter input",
      |       "minString": "",
      |       "maxString": "",
      |       "width": 1,
      |       "dataType": 0,
      |       "signalType": 0,
      |       "createSignal": false,
      |       "outputName": "LowVoltageBatterySOC[0_1]",
      |       "generateSignalAccessBlock": false,
      |       "accessId": "$(parentId).$(blockName).$(outputName)"
      |     }
      |   ]
      | }
      mask prompts: NeedsUpdate "Specify, if subsystem content needs to be updated"; SignalInfo "Signal Info (json)"
      mask help: DYNA4 Interface Block Version 4.6
      mask init:
      | blockName = get_param(gcbh, 'Name');
      | parentId = DYNA4.ModelHandling.AccessID.getFromHierarchy(gcbh);
      | TD.InterfaceBlock.ModelCallbacks.GenerateContent(gcb);
      settings: DeleteFcn=TD.InterfaceBlock.ModelCallbacks.CloseGUI( gcbh );  NameChangeFcn=TD.InterfaceBlock.ModelCallbacks.BlockRenamedHandler(gcbh);  OpenFcn=TD.InterfaceBlock.ModelCallbacks.OpenGUI( gcbh );  CloseFcn=TD.InterfaceBlock.ModelCallbacks.CloseGUI( gcbh );
      mask Display:
      | image('InterfaceBlock.png','center');
      | port_label('input',1, 'LowVoltageBatteryVoltage[V]');
      | port_label('input',2, 'LowVoltageBatterySOC[0_1]');
      | port_label('output',1, 'LowVoltageBattery');
  LowVoltageBatteryVoltage : LookupTableModules/ConstantVoltage  DATA_NODE=MDL.Vehicle.ElectricalSystem.LowVoltageBatteryVoltage  ConstVoltage=MDL.Vehicle.ElectricalSystem.LowVoltageBatteryVoltage.Voltage
  Terminator_{1..4} (4 alike) : Terminator
  TraceMarker : UtilitiesLibrary/DYNA4 Trace Marker  Tag=DYNA4_TRACE_MARKER  SettingType=Standard  PrefixModelBlockID=on  PrefixRootSignalName=off  NamePattern='$(modelBlockID).$(rootSignalName)'
  ElectricalSystem : Outport  VectorParamsAs1DForOutWhenUnconnected=off
  wires:
  ElectricalSystemOutput/1(ElectricalSystem___UNIQUE_1) -> ElectricalSystem/1, TraceMarker/1
  fromAuxiliaries/1 -> Terminator_4/1
  fromDrivetrain/1 -> Terminator_2/1
  fromCTRL/1 -> Terminator_3/1
  fromEngine/1 -> Terminator_1/1
  LowVoltageBatteryVoltage/1 -> ElectricalSystemOutput/3(GeneratorVoltage[V]___UNIQUE_1), ElectricalSystemOutput/2(StarterVoltage[V]___UNIQUE_1), LowVoltageBatteryOutput/1(LowVoltageBatteryVoltage[V]___UNIQUE_1)
  LowVoltageBatteryInitialSOC/1 -> LowVoltageBatteryOutput/2(LowVoltageBatterySOC[0_1]___UNIQUE_1)
  LowVoltageBatteryOutput/1(LowVoltageBattery___UNIQUE_1) -> ElectricalSystemOutput/1(LowVoltageBattery___UNIQUE_1)
